simulink model "lab2_2"  (Simulink 7.3)
settings: Solver=ode45  StartTime=0.0  StopTime=1  RelTol=1e-3
settings Model: Creator=student  LastModifiedBy=student

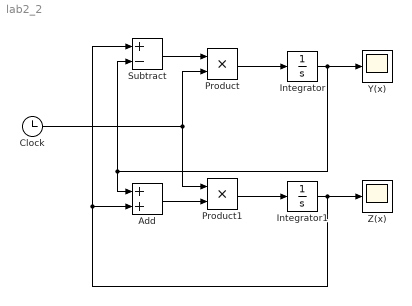
== system lab2_2 ==
  Add : Sum  OutDataType=fixdt(1, 16)  OutScaling=2^-10
  Clock : Clock
      settings: Decimation=10
  Integrator : Integrator  InitialCondition=1
  Integrator1 : Integrator  InitialCondition=1
  Product : Product  OutDataType=fixdt(1, 16)  OutScaling=2^0  RndMeth=Zero
  Product1 : Product  OutDataType=fixdt(1, 16)  OutScaling=2^0  RndMeth=Zero
  Subtract : Sum  Inputs=+-  OutDataType=fixdt(1, 16)  OutScaling=2^-10
  Y(x) : Scope
  Z(x) : Scope
  wires:
  Subtract/1 -> Product/1
  Clock/1 -> Product/2, Product1/1
  Add/1 -> Product1/2
  Product/1 -> Integrator/1
  Product1/1 -> Integrator1/1
  Integrator1/1 -> Subtract/1, Add/2, Z(x)/1
  Integrator/1 -> Add/1, Subtract/2, Y(x)/1
